simulink subsystem "Final_Project_PreRemoveOutputAdapter_20260527_143352"  (R2024a)
settings: Solver=VariableStepAuto  StartTime=0.0  StopTime=10.0  RelTol=1e-3
libraries: CarMaker4SL x42
settings Model: Creator=junho.lee  LastModifiedBy=hajin

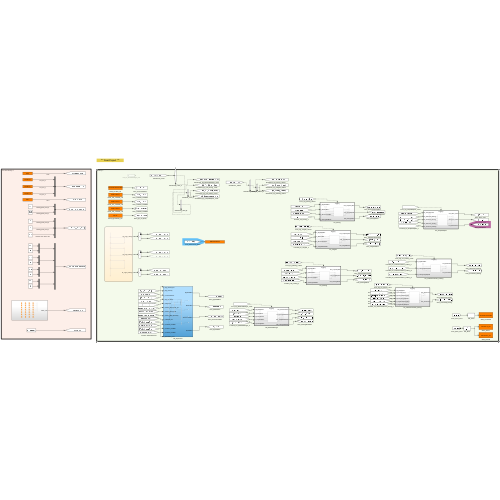
[thumbnail: Simulink's stored preview of the top-level diagram]
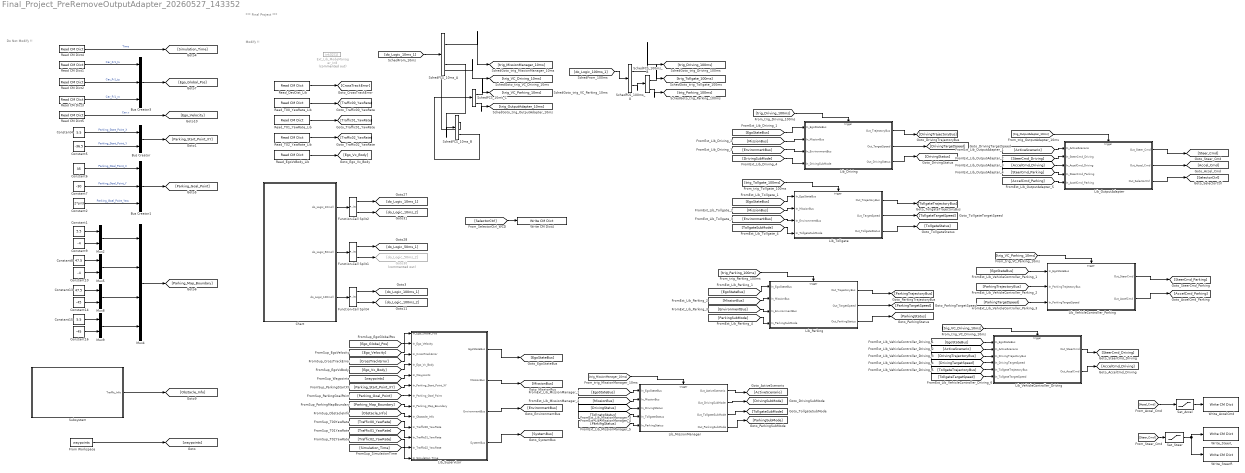
== system Final_Project_PreRemoveOutputAdapter_20260527_143352 ==
  note: Do Not Modify !!
  note: *** Final Project ***
  note: Modify !!
  Bus Creator : BusCreator  Inputs=2
  Bus Creator1 : BusCreator  Inputs=3
  Bus Creator3 : BusCreator  Inputs=3
  Chart : Stateflow chart  TreatAsAtomicUnit=on
  Constant1 : Constant  Value=5.5
  Constant10 : Constant  Value=-4
  Constant13 : Constant  Value=47.5
  Constant14 : Constant  Value=-45
  Constant15 : Constant  Value=5.5
  Constant16 : Constant  Value=-45
  Constant2 : Constant  Value=2*pi/3
  Constant4 : Constant  Value=5.5
  Constant5 : Constant  Value=-36.5
  Constant6 : Constant  Value=35
  Constant7 : Constant  Value=-30
  Constant8 : Constant  Value=47.5
  Constant9 : Constant  Value=-4
  Ext_Lib_ModeManager_In8 : Constant  Commented=on  Value=int32(1)  OutDataTypeStr=int32
  From Workspace : FromWorkspace  VariableName=waypoints
  Function-Call Split1 : FunctionCallSplit  IconShape=distinctive  NumOutputPorts=2  OutputPortLayout=default
  Function-Call Split2 : FunctionCallSplit  IconShape=distinctive  NumOutputPorts=2  OutputPortLayout=default
  Function-Call Split4 : FunctionCallSplit  IconShape=distinctive  NumOutputPorts=2  OutputPortLayout=default
  Goto30 : Goto  Commented=on  GotoTag=do_Logic_50ms_2
  Lib_Driving : Subsystem
  Lib_MissionManager : Subsystem
  Lib_OutputAdapter : Subsystem
  Lib_Parking : Subsystem
  Lib_Supervisor : Subsystem
  Lib_Tollgate : Subsystem
  Lib_VehicleController_Driving : Subsystem
  Lib_VehicleController_Parking : Subsystem
  Mux{2,5,8..9} (4 alike) : Mux  Inputs=2
  Mux4 : Mux
  Read CM Dict1 : CarMaker4SL/Read CM Dict  xname=Car.Fr1.tx  xsync=off  xstime=Inherited
  Read CM Dict2 : CarMaker4SL/Read CM Dict  xname=Car.Fr1.ty  xsync=off  xstime=Inherited
  Read CM Dict3 : CarMaker4SL/Read CM Dict  xname=Car.Fr1.rz  xsync=off  xstime=Inherited
  Read CM Dict4 : CarMaker4SL/Read CM Dict  xname=Time  xsync=off  xstime=Inherited
  Read CM Dict5 : CarMaker4SL/Read CM Dict  xname=Car.v  xsync=off  xstime=Inherited
  Read_DevDist_Lib : CarMaker4SL/Read CM Dict  xname=Car.Road.Path.DevDist  xsync=off  xstime=Inherited
  Read_EgoVxBody_Lib : CarMaker4SL/Read CM Dict  xname=Car.vx  xsync=off  xstime=Inherited
  Read_T00_YawRate_Lib : CarMaker4SL/Read CM Dict  xname=Traffic.T00.rzv  xsync=off  xstime=Inherited
  Read_T01_YawRate_Lib : CarMaker4SL/Read CM Dict  xname=Traffic.T01.rzv  xsync=off  xstime=Inherited
  Read_T02_YawRate_Lib : CarMaker4SL/Read CM Dict  xname=Traffic.T02.rzv  xsync=off  xstime=Inherited
  Sat_Accel : Saturate  UpperLimit=3.0  LowerLimit=-5.0
  Sat_Steer : Saturate  UpperLimit=pi/6  LowerLimit=-pi/6
  SchedFCS_100ms_A : FunctionCallSplit  NumOutputPorts=2
  SchedFCS_100ms_B : FunctionCallSplit  NumOutputPorts=2
  SchedFCS_10ms_A : FunctionCallSplit  NumOutputPorts=2
  SchedFCS_10ms_B : FunctionCallSplit  NumOutputPorts=2
  SchedFCS_10ms_C : FunctionCallSplit  NumOutputPorts=2
  Subsystem : Subsystem
  Write CM Dict4 : CarMaker4SL/Write CM Dict  xname=DM.SelectorCtrl  xsync=off
  Write_AccelCmd : CarMaker4SL/Write CM Dict  xname=AccelCtrl.DesiredAx  xsync=off
  Write_SteerL : CarMaker4SL/Write CM Dict  xname=Car.CFL.rz_ext  xsync=off
  Write_SteerR : CarMaker4SL/Write CM Dict  xname=Car.CFR.rz_ext  xsync=off
  wires:
  Constant13/1 -> Mux8/1
  Subsystem/1(Traffic_Info) -> [Obstacle_Info]
  Read CM Dict1/1 -> Bus Creator3/1  "Car_Fr1_tx"
  Read CM Dict3/1 -> Bus Creator3/3  "Car_Fr1_rz"
  Constant4/1 -> Bus Creator/1  "Parking_Start_Point_X"
  Chart/2(do_Logic_50ms()) -> Function-Call Split1/1
  Function-Call Split2/1 -> [do_Logic_10ms_1]
  Function-Call Split1/2 -> Goto30/1
  Read CM Dict4/1 -> [Simulation_Time]  "Time"
  Constant9/1 -> Mux2/2
  Bus Creator1/1 -> [Parking_Goal_Point]
  Mux8/1 -> Mux4/3
  Constant6/1 -> Bus Creator1/1  "Parking_Goal_Point_X"
  Constant1/1 -> Mux2/1
  Constant16/1 -> Mux9/2
  Read CM Dict2/1 -> Bus Creator3/2  "Car_Fr1_ty"
  Function-Call Split1/1 -> [do_Logic_50ms_1]
  Constant5/1 -> Bus Creator/2  "Parking_Start_Point_Y"
  Chart/1(do_Logic_10ms()) -> Function-Call Split2/1
  Constant7/1 -> Bus Creator1/2  "Parking_Goal_Point_Y"
  Read CM Dict5/1 -> [Ego_Velocity]  "Car.v"
  Constant15/1 -> Mux9/1
  Constant10/1 -> Mux5/2
  Bus Creator3/1 -> [Ego_Global_Pos]
  Constant14/1 -> Mux8/2
  Function-Call Split2/2 -> [do_Logic_10ms_2]
  Bus Creator/1 -> [Parking_Start_Point_XY]
  Mux9/1 -> Mux4/4
  Mux2/1 -> Mux4/1
  Mux4/1 -> [Parking_Map_Boundary]
  Constant8/1 -> Mux5/1
  Constant2/1 -> Bus Creator1/3  "Parking_Goal_Point_Yaw"
  Mux5/1 -> Mux4/2
  Chart/3(do_Logic_100ms()) -> Function-Call Split4/1
  Function-Call Split4/1 -> [do_Logic_100ms_1]
  Function-Call Split4/2 -> [do_Logic_100ms_2]
  From Workspace/1 -> [waypoints]
  [Accel_Cmd] -> Sat_Accel/1
  Sat_Accel/1 -> Write_AccelCmd/1
  [Steer_Cmd] -> Sat_Steer/1
  Sat_Steer/1 -> Write_SteerR/1, Write_SteerL/1
  Read_DevDist_Lib/1 -> [CrossTrackError]
  Read_T00_YawRate_Lib/1 -> [Traffic00_YawRate]
  Read_T01_YawRate_Lib/1 -> [Traffic01_YawRate]
  Read_T02_YawRate_Lib/1 -> [Traffic02_YawRate]
  Read_EgoVxBody_Lib/1 -> [Ego_Vx_Body]
  [Ego_Global_Pos] -> Lib_Supervisor/1(In_Ego_Global_Pos)
  [Ego_Velocity] -> Lib_Supervisor/2(In_Ego_Velocity)
  [CrossTrackError] -> Lib_Supervisor/3(In_CrossTrackError)
  [Ego_Vx_Body] -> Lib_Supervisor/4(In_Ego_Vx_Body)
  [waypoints] -> Lib_Supervisor/5(In_Waypoints)
  [Parking_Start_Point_XY] -> Lib_Supervisor/6(In_Parking_Start_Point_XY)
  [Parking_Goal_Point] -> Lib_Supervisor/7(In_Parking_Goal_Point)
  [Parking_Map_Boundary] -> Lib_Supervisor/8(In_Parking_Map_Boundary)
  [Obstacle_Info] -> Lib_Supervisor/9(In_Obstacle_Info)
  [Traffic00_YawRate] -> Lib_Supervisor/10(In_Traffic00_YawRate)
  [Traffic01_YawRate] -> Lib_Supervisor/11(In_Traffic01_YawRate)
  [Traffic02_YawRate] -> Lib_Supervisor/12(In_Traffic02_YawRate)
  [Simulation_Time] -> Lib_Supervisor/13(In_Simulation_Time)
  Lib_Supervisor/1(EgoStateBus) -> [EgoStateBus]
  Lib_Supervisor/2(MissionBus) -> [MissionBus]
  Lib_Supervisor/3(EnvironmentBus) -> [EnvironmentBus]
  Lib_Supervisor/4(SystemBus) -> [SystemBus]
  Lib_MissionManager/1(Out_ActiveScenario) -> [ActiveScenario]
  Lib_MissionManager/2(Out_DrivingSubMode) -> [DrivingSubMode]
  Lib_MissionManager/3(Out_TollgateSubMode) -> [TollgateSubMode]
  Lib_MissionManager/4(Out_ParkingSubMode) -> [ParkingSubMode]
  Lib_Driving/1(Out_TrajectoryBus) -> [DrivingTrajectoryBus]
  Lib_Driving/2(Out_TargetSpeed) -> [DrivingTargetSpeed]
  Lib_Driving/3(Out_DrivingStatus) -> [DrivingStatus]
  Lib_Tollgate/1(Out_TrajectoryBus) -> [TollgateTrajectoryBus]
  Lib_Tollgate/2(Out_TargetSpeed) -> [TollgateTargetSpeed]
  Lib_Tollgate/3(Out_TollgateStatus) -> [TollgateStatus]
  Lib_Parking/1(Out_TrajectoryBus) -> [ParkingTrajectoryBus]
  Lib_Parking/2(Out_TargetSpeed) -> [ParkingTargetSpeed]
  Lib_Parking/3(Out_ParkingStatus) -> [ParkingStatus]
  Lib_VehicleController_Driving/1(Out_SteerCmd) -> [SteerCmd_Driving]
  Lib_VehicleController_Driving/2(Out_AccelCmd) -> [AccelCmd_Driving]
  Lib_VehicleController_Parking/1(Out_SteerCmd) -> [SteerCmd_Parking]
  Lib_VehicleController_Parking/2(Out_AccelCmd) -> [AccelCmd_Parking]
  Lib_OutputAdapter/1(Out_Steer_Cmd) -> [Steer_Cmd]
  Lib_OutputAdapter/2(Out_Accel_Cmd) -> [Accel_Cmd]
  Lib_OutputAdapter/3(Out_SelectorCtrl) -> [SelectorCtrl]
  [EgoStateBus] -> Lib_MissionManager/1(In_EgoStateBus)
  [MissionBus] -> Lib_MissionManager/2(In_MissionBus)
  [DrivingStatus] -> Lib_MissionManager/3(In_DrivingStatus)
  [TollgateStatus] -> Lib_MissionManager/4(In_TollgateStatus)
  [ParkingStatus] -> Lib_MissionManager/5(In_ParkingStatus)
  [EgoStateBus] -> Lib_Driving/1(In_EgoStateBus)
  [MissionBus] -> Lib_Driving/2(In_MissionBus)
  [EnvironmentBus] -> Lib_Driving/3(In_EnvironmentBus)
  [DrivingSubMode] -> Lib_Driving/4(In_DrivingSubMode)
  [EgoStateBus] -> Lib_Tollgate/1(In_EgoStateBus)
  [MissionBus] -> Lib_Tollgate/2(In_MissionBus)
  [EnvironmentBus] -> Lib_Tollgate/3(In_EnvironmentBus)
  [TollgateSubMode] -> Lib_Tollgate/4(In_TollgateSubMode)
  [EgoStateBus] -> Lib_Parking/1(In_EgoStateBus)
  [MissionBus] -> Lib_Parking/2(In_MissionBus)
  [EnvironmentBus] -> Lib_Parking/3(In_EnvironmentBus)
  [ParkingSubMode] -> Lib_Parking/4(In_ParkingSubMode)
  [EgoStateBus] -> Lib_VehicleController_Driving/1(In_EgoStateBus)
  [ActiveScenario] -> Lib_VehicleController_Driving/2(In_ActiveScenario)
  [DrivingTrajectoryBus] -> Lib_VehicleController_Driving/3(In_DrivingTrajectoryBus)
  [DrivingTargetSpeed] -> Lib_VehicleController_Driving/4(In_DrivingTargetSpeed)
  [TollgateTrajectoryBus] -> Lib_VehicleController_Driving/5(In_TollgateTrajectoryBus)
  [TollgateTargetSpeed] -> Lib_VehicleController_Driving/6(In_TollgateTargetSpeed)
  [EgoStateBus] -> Lib_VehicleController_Parking/1(In_EgoStateBus)
  [ParkingTrajectoryBus] -> Lib_VehicleController_Parking/2(In_ParkingTrajectoryBus)
  [ParkingTargetSpeed] -> Lib_VehicleController_Parking/3(In_ParkingTargetSpeed)
  [ActiveScenario] -> Lib_OutputAdapter/1(In_ActiveScenario)
  [SteerCmd_Driving] -> Lib_OutputAdapter/2(In_SteerCmd_Driving)
  [AccelCmd_Driving] -> Lib_OutputAdapter/3(In_AccelCmd_Driving)
  [SteerCmd_Parking] -> Lib_OutputAdapter/4(In_SteerCmd_Parking)
  [AccelCmd_Parking] -> Lib_OutputAdapter/5(In_AccelCmd_Parking)
  [do_Logic_10ms_1] -> SchedFCS_10ms_A/1
  SchedFCS_10ms_A/1 -> [trig_MissionManager_10ms]
  SchedFCS_10ms_A/2 -> SchedFCS_10ms_B/1
  SchedFCS_10ms_B/1 -> [trig_VC_Driving_10ms]
  SchedFCS_10ms_B/2 -> SchedFCS_10ms_C/1
  SchedFCS_10ms_C/1 -> [trig_VC_Parking_10ms]
  SchedFCS_10ms_C/2 -> [trig_OutputAdapter_10ms]
  [do_Logic_100ms_1] -> SchedFCS_100ms_A/1
  SchedFCS_100ms_A/1 -> [trig_Driving_100ms]
  SchedFCS_100ms_A/2 -> SchedFCS_100ms_B/1
  SchedFCS_100ms_B/1 -> [trig_Tollgate_100ms]
  SchedFCS_100ms_B/2 -> [trig_Parking_100ms]
  [trig_MissionManager_10ms] -> Lib_MissionManager/Trigger
  [trig_VC_Driving_10ms] -> Lib_VehicleController_Driving/Trigger
  [trig_VC_Parking_10ms] -> Lib_VehicleController_Parking/Trigger
  [trig_OutputAdapter_10ms] -> Lib_OutputAdapter/Trigger
  [trig_Driving_100ms] -> Lib_Driving/Trigger
  [trig_Tollgate_100ms] -> Lib_Tollgate/Trigger
  [trig_Parking_100ms] -> Lib_Parking/Trigger
  [SelectorCtrl] -> Write CM Dict4/1

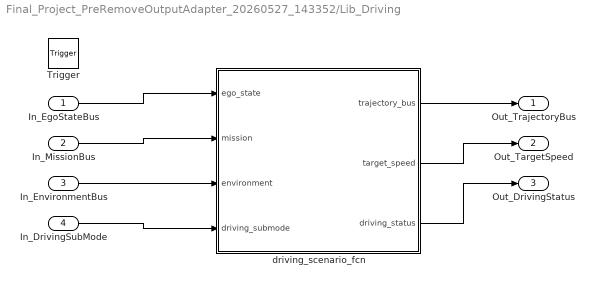
== system Final_Project_PreRemoveOutputAdapter_20260527_143352/Lib_Driving ==
  In_EgoStateBus : Inport
  In_MissionBus : Inport  Port=2
  In_EnvironmentBus : Inport  Port=3
  In_DrivingSubMode : Inport  Port=4
  Trigger : TriggerPort  TriggerType=function-call  VariantControl=(inherit)
  driving_scenario_fcn : MATLAB Function  TreatAsAtomicUnit=on
  Out_TrajectoryBus : Outport
  Out_TargetSpeed : Outport  Port=2
  Out_DrivingStatus : Outport  Port=3
  wires:
  In_EgoStateBus/1 -> driving_scenario_fcn/1(ego_state)
  In_MissionBus/1 -> driving_scenario_fcn/2(mission)
  In_EnvironmentBus/1 -> driving_scenario_fcn/3(environment)
  In_DrivingSubMode/1 -> driving_scenario_fcn/4(driving_submode)
  driving_scenario_fcn/1(trajectory_bus) -> Out_TrajectoryBus/1
  driving_scenario_fcn/2(target_speed) -> Out_TargetSpeed/1
  driving_scenario_fcn/3(driving_status) -> Out_DrivingStatus/1

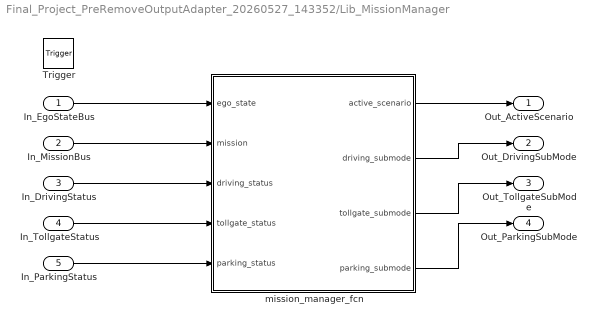
== system Final_Project_PreRemoveOutputAdapter_20260527_143352/Lib_MissionManager ==
  In_EgoStateBus : Inport
  In_MissionBus : Inport  Port=2
  In_DrivingStatus : Inport  Port=3
  In_TollgateStatus : Inport  Port=4
  In_ParkingStatus : Inport  Port=5
  Trigger : TriggerPort  TriggerType=function-call  VariantControl=(inherit)
  mission_manager_fcn : MATLAB Function  TreatAsAtomicUnit=on
  Out_ActiveScenario : Outport
  Out_DrivingSubMode : Outport  Port=2
  Out_TollgateSubMode : Outport  Port=3
  Out_ParkingSubMode : Outport  Port=4
  wires:
  In_EgoStateBus/1 -> mission_manager_fcn/1(ego_state)
  In_MissionBus/1 -> mission_manager_fcn/2(mission)
  In_DrivingStatus/1 -> mission_manager_fcn/3(driving_status)
  In_TollgateStatus/1 -> mission_manager_fcn/4(tollgate_status)
  In_ParkingStatus/1 -> mission_manager_fcn/5(parking_status)
  mission_manager_fcn/1(active_scenario) -> Out_ActiveScenario/1
  mission_manager_fcn/2(driving_submode) -> Out_DrivingSubMode/1
  mission_manager_fcn/3(tollgate_submode) -> Out_TollgateSubMode/1
  mission_manager_fcn/4(parking_submode) -> Out_ParkingSubMode/1

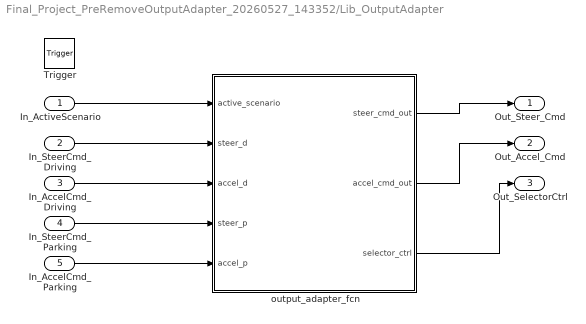
== system Final_Project_PreRemoveOutputAdapter_20260527_143352/Lib_OutputAdapter ==
  In_ActiveScenario : Inport
  In_SteerCmd_Driving : Inport  Port=2
  In_AccelCmd_Driving : Inport  Port=3
  In_SteerCmd_Parking : Inport  Port=4
  In_AccelCmd_Parking : Inport  Port=5
  Trigger : TriggerPort  TriggerType=function-call  VariantControl=(inherit)
  output_adapter_fcn : MATLAB Function  TreatAsAtomicUnit=on
  Out_Steer_Cmd : Outport
  Out_Accel_Cmd : Outport  Port=2
  Out_SelectorCtrl : Outport  Port=3
  wires:
  In_ActiveScenario/1 -> output_adapter_fcn/1(active_scenario)
  In_SteerCmd_Driving/1 -> output_adapter_fcn/2(steer_d)
  In_AccelCmd_Driving/1 -> output_adapter_fcn/3(accel_d)
  In_SteerCmd_Parking/1 -> output_adapter_fcn/4(steer_p)
  In_AccelCmd_Parking/1 -> output_adapter_fcn/5(accel_p)
  output_adapter_fcn/1(steer_cmd_out) -> Out_Steer_Cmd/1
  output_adapter_fcn/2(accel_cmd_out) -> Out_Accel_Cmd/1
  output_adapter_fcn/3(selector_ctrl) -> Out_SelectorCtrl/1

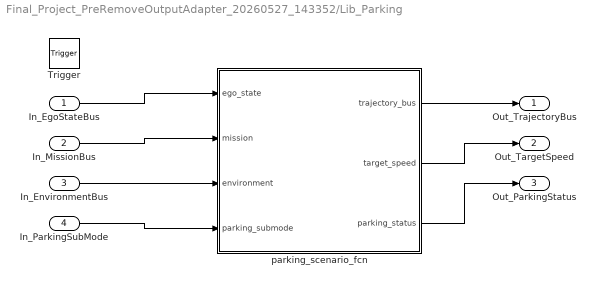
== system Final_Project_PreRemoveOutputAdapter_20260527_143352/Lib_Parking ==
  In_EgoStateBus : Inport
  In_MissionBus : Inport  Port=2
  In_EnvironmentBus : Inport  Port=3
  In_ParkingSubMode : Inport  Port=4
  Trigger : TriggerPort  TriggerType=function-call  VariantControl=(inherit)
  parking_scenario_fcn : MATLAB Function  TreatAsAtomicUnit=on
  Out_TrajectoryBus : Outport
  Out_TargetSpeed : Outport  Port=2
  Out_ParkingStatus : Outport  Port=3
  wires:
  In_EgoStateBus/1 -> parking_scenario_fcn/1(ego_state)
  In_MissionBus/1 -> parking_scenario_fcn/2(mission)
  In_EnvironmentBus/1 -> parking_scenario_fcn/3(environment)
  In_ParkingSubMode/1 -> parking_scenario_fcn/4(parking_submode)
  parking_scenario_fcn/1(trajectory_bus) -> Out_TrajectoryBus/1
  parking_scenario_fcn/2(target_speed) -> Out_TargetSpeed/1
  parking_scenario_fcn/3(parking_status) -> Out_ParkingStatus/1

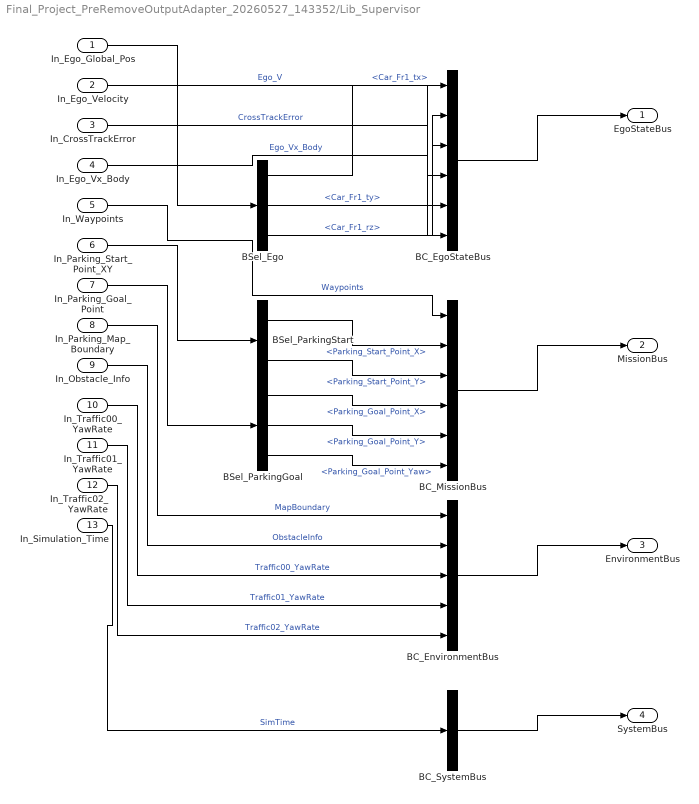
== system Final_Project_PreRemoveOutputAdapter_20260527_143352/Lib_Supervisor ==
  In_Ego_Global_Pos : Inport
  In_Ego_Velocity : Inport  Port=2
  In_CrossTrackError : Inport  Port=3
  In_Ego_Vx_Body : Inport  Port=4
  In_Waypoints : Inport  Port=5
  In_Parking_Start_Point_XY : Inport  Port=6
  In_Parking_Goal_Point : Inport  Port=7
  In_Parking_Map_Boundary : Inport  Port=8
  In_Obstacle_Info : Inport  Port=9
  In_Traffic00_YawRate : Inport  Port=10
  In_Traffic01_YawRate : Inport  Port=11
  In_Traffic02_YawRate : Inport  Port=12
  In_Simulation_Time : Inport  Port=13
  BC_EgoStateBus : BusCreator  Inputs=6
  BC_EnvironmentBus : BusCreator  Inputs=5
  BC_MissionBus : BusCreator  Inputs=6
  BC_SystemBus : BusCreator  Inputs=1
  BSel_Ego : BusSelector  OutputSignals=Car_Fr1_tx,Car_Fr1_ty,Car_Fr1_rz
  BSel_ParkingGoal : BusSelector  OutputSignals=Parking_Goal_Point_X,Parking_Goal_Point_Y,Parking_Goal_Point_Yaw
  BSel_ParkingStart : BusSelector  OutputSignals=Parking_Start_Point_X,Parking_Start_Point_Y
  EgoStateBus : Outport
  MissionBus : Outport  Port=2
  EnvironmentBus : Outport  Port=3
  SystemBus : Outport  Port=4
  wires:
  In_Ego_Global_Pos/1 -> BSel_Ego/1
  In_Parking_Start_Point_XY/1 -> BSel_ParkingStart/1
  In_Parking_Goal_Point/1 -> BSel_ParkingGoal/1
  BSel_Ego/1 -> BC_EgoStateBus/1  "<Car_Fr1_tx>"
  BSel_Ego/2 -> BC_EgoStateBus/2  "<Car_Fr1_ty>"
  BSel_Ego/3 -> BC_EgoStateBus/3  "<Car_Fr1_rz>"
  In_Ego_Velocity/1 -> BC_EgoStateBus/4  "Ego_V"
  In_CrossTrackError/1 -> BC_EgoStateBus/5  "CrossTrackError"
  In_Ego_Vx_Body/1 -> BC_EgoStateBus/6  "Ego_Vx_Body"
  In_Waypoints/1 -> BC_MissionBus/1  "Waypoints"
  BSel_ParkingStart/1 -> BC_MissionBus/2  "<Parking_Start_Point_X>"
  BSel_ParkingStart/2 -> BC_MissionBus/3  "<Parking_Start_Point_Y>"
  BSel_ParkingGoal/1 -> BC_MissionBus/4  "<Parking_Goal_Point_X>"
  BSel_ParkingGoal/2 -> BC_MissionBus/5  "<Parking_Goal_Point_Y>"
  BSel_ParkingGoal/3 -> BC_MissionBus/6  "<Parking_Goal_Point_Yaw>"
  In_Parking_Map_Boundary/1 -> BC_EnvironmentBus/1  "MapBoundary"
  In_Obstacle_Info/1 -> BC_EnvironmentBus/2  "ObstacleInfo"
  In_Traffic00_YawRate/1 -> BC_EnvironmentBus/3  "Traffic00_YawRate"
  In_Traffic01_YawRate/1 -> BC_EnvironmentBus/4  "Traffic01_YawRate"
  In_Traffic02_YawRate/1 -> BC_EnvironmentBus/5  "Traffic02_YawRate"
  In_Simulation_Time/1 -> BC_SystemBus/1  "SimTime"
  BC_EgoStateBus/1 -> EgoStateBus/1
  BC_MissionBus/1 -> MissionBus/1
  BC_EnvironmentBus/1 -> EnvironmentBus/1
  BC_SystemBus/1 -> SystemBus/1

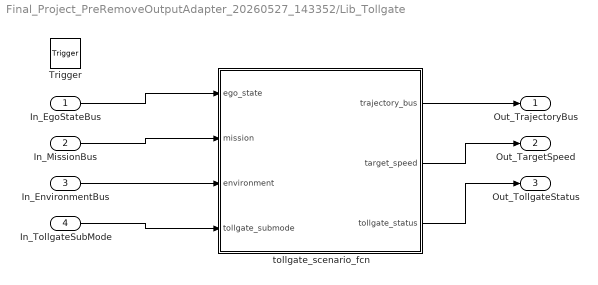
== system Final_Project_PreRemoveOutputAdapter_20260527_143352/Lib_Tollgate ==
  In_EgoStateBus : Inport
  In_MissionBus : Inport  Port=2
  In_EnvironmentBus : Inport  Port=3
  In_TollgateSubMode : Inport  Port=4
  Trigger : TriggerPort  TriggerType=function-call  VariantControl=(inherit)
  tollgate_scenario_fcn : MATLAB Function  TreatAsAtomicUnit=on
  Out_TrajectoryBus : Outport
  Out_TargetSpeed : Outport  Port=2
  Out_TollgateStatus : Outport  Port=3
  wires:
  In_EgoStateBus/1 -> tollgate_scenario_fcn/1(ego_state)
  In_MissionBus/1 -> tollgate_scenario_fcn/2(mission)
  In_EnvironmentBus/1 -> tollgate_scenario_fcn/3(environment)
  In_TollgateSubMode/1 -> tollgate_scenario_fcn/4(tollgate_submode)
  tollgate_scenario_fcn/1(trajectory_bus) -> Out_TrajectoryBus/1
  tollgate_scenario_fcn/2(target_speed) -> Out_TargetSpeed/1
  tollgate_scenario_fcn/3(tollgate_status) -> Out_TollgateStatus/1

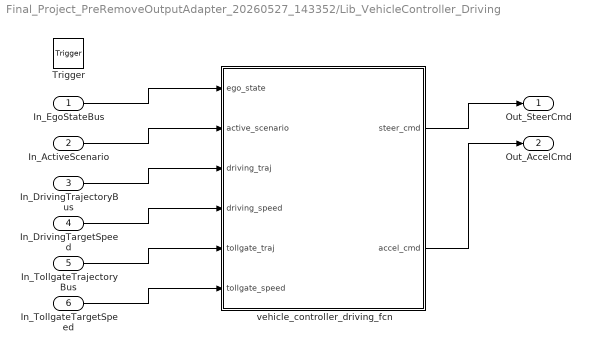
== system Final_Project_PreRemoveOutputAdapter_20260527_143352/Lib_VehicleController_Driving ==
  In_EgoStateBus : Inport
  In_ActiveScenario : Inport  Port=2
  In_DrivingTrajectoryBus : Inport  Port=3
  In_DrivingTargetSpeed : Inport  Port=4
  In_TollgateTrajectoryBus : Inport  Port=5
  In_TollgateTargetSpeed : Inport  Port=6
  Trigger : TriggerPort  TriggerType=function-call  VariantControl=(inherit)
  vehicle_controller_driving_fcn : MATLAB Function  TreatAsAtomicUnit=on
  Out_SteerCmd : Outport
  Out_AccelCmd : Outport  Port=2
  wires:
  In_EgoStateBus/1 -> vehicle_controller_driving_fcn/1(ego_state)
  In_ActiveScenario/1 -> vehicle_controller_driving_fcn/2(active_scenario)
  In_DrivingTrajectoryBus/1 -> vehicle_controller_driving_fcn/3(driving_traj)
  In_DrivingTargetSpeed/1 -> vehicle_controller_driving_fcn/4(driving_speed)
  In_TollgateTrajectoryBus/1 -> vehicle_controller_driving_fcn/5(tollgate_traj)
  In_TollgateTargetSpeed/1 -> vehicle_controller_driving_fcn/6(tollgate_speed)
  vehicle_controller_driving_fcn/1(steer_cmd) -> Out_SteerCmd/1
  vehicle_controller_driving_fcn/2(accel_cmd) -> Out_AccelCmd/1

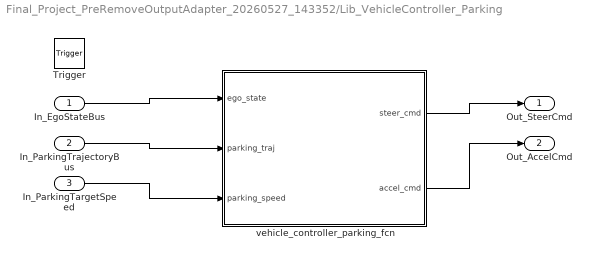
== system Final_Project_PreRemoveOutputAdapter_20260527_143352/Lib_VehicleController_Parking ==
  In_EgoStateBus : Inport
  In_ParkingTrajectoryBus : Inport  Port=2
  In_ParkingTargetSpeed : Inport  Port=3
  Trigger : TriggerPort  TriggerType=function-call  VariantControl=(inherit)
  vehicle_controller_parking_fcn : MATLAB Function  TreatAsAtomicUnit=on
  Out_SteerCmd : Outport
  Out_AccelCmd : Outport  Port=2
  wires:
  In_EgoStateBus/1 -> vehicle_controller_parking_fcn/1(ego_state)
  In_ParkingTrajectoryBus/1 -> vehicle_controller_parking_fcn/2(parking_traj)
  In_ParkingTargetSpeed/1 -> vehicle_controller_parking_fcn/3(parking_speed)
  vehicle_controller_parking_fcn/1(steer_cmd) -> Out_SteerCmd/1
  vehicle_controller_parking_fcn/2(accel_cmd) -> Out_AccelCmd/1

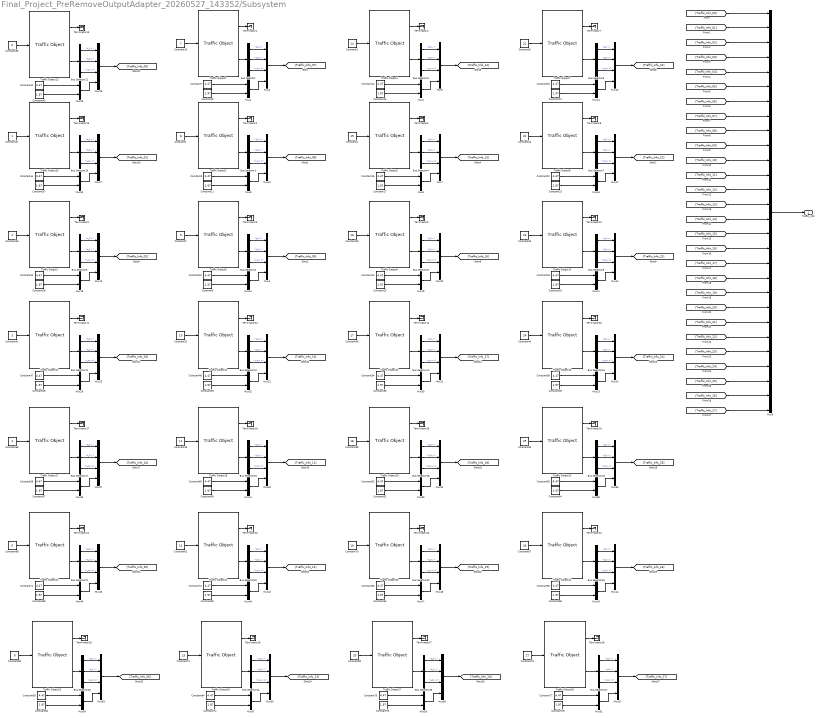
== system Final_Project_PreRemoveOutputAdapter_20260527_143352/Subsystem ==
  Bus Selector{,1..27} (28 alike) : BusSelector  OutputSignals=t_0 x,t_0 y,r_zyx z
  Constant1 : Constant  Value=8
  Constant10 : Constant  Value=7
  Constant{5,8,11,13,15,17,19,21,23,28,33,35,37,39,43,45,50,52,54,57,62,64,66,69,74,76,78,81} (28 alike) : Constant  Value=1.97
  Constant{7,9,12,14,16,18,20,22,30..31,34,38,42,44,47..48,51,53,59..60,63,65,71..72,75,77,83..84} (28 alike) : Constant  Value=4.47
  Constant2 : Constant  Value=9
  Constant24 : Constant  Value=22
  Constant25 : Constant  Value=23
  Constant26 : Constant  Value=2
  Constant27 : Constant
  Constant29 : Constant  Value=16
  Constant3 : Constant  Value=14
  Constant32 : Constant  Value=10
  Constant36 : Constant  Value=0
  Constant4 : Constant  Value=15
  Constant40 : Constant  Value=24
  Constant41 : Constant  Value=3
  Constant46 : Constant  Value=17
  Constant49 : Constant  Value=11
  Constant55 : Constant  Value=25
  Constant56 : Constant  Value=4
  Constant58 : Constant  Value=18
  Constant6 : Constant  Value=21
  Constant61 : Constant  Value=12
  Constant67 : Constant  Value=26
  Constant68 : Constant  Value=5
  Constant70 : Constant  Value=19
  Constant73 : Constant  Value=13
  Constant79 : Constant  Value=27
  Constant80 : Constant  Value=6
  Constant82 : Constant  Value=20
  Mux{1,4,6,8,11,14,16,18..19,21,23,26,28,30,32..33,35,38..39,41,43,46..47,49,51,54..55,57} (28 alike) : Mux  Inputs=2
  Mux{2..3,5,7,10,12..13,15,17,20,22,24..25,27,29,31,34,36..37,40,42,44..45,48,50,52..53,56} (28 alike) : Mux
  Mux9 : Mux  Inputs=28
  Terminator{1..28} (28 alike) : Terminator
  Traffic Object1 : CarMaker4SL/Traffic Object  xname=T07  ximode=Traffic Id  xstime=Inherited
      settings: SourceProductName=CarMaker4SL
  Traffic Object10 : CarMaker4SL/Traffic Object  xname=T23  ximode=Traffic Id  xstime=Inherited
      settings: SourceProductName=CarMaker4SL
  Traffic Object11 : CarMaker4SL/Traffic Object  xname=T03  ximode=Traffic Id  xstime=Inherited
      settings: SourceProductName=CarMaker4SL
  Traffic Object12 : CarMaker4SL/Traffic Object  xname=T10  ximode=Traffic Id  xstime=Inherited
      settings: SourceProductName=CarMaker4SL
  Traffic Object13 : CarMaker4SL/Traffic Object  xname=T00  ximode=Traffic Id  xstime=Inherited
      settings: SourceProductName=CarMaker4SL
  Traffic Object14 : CarMaker4SL/Traffic Object  xname=T17  ximode=Traffic Id  xstime=Inherited
      settings: SourceProductName=CarMaker4SL
  Traffic Object15 : CarMaker4SL/Traffic Object  xname=T01  ximode=Traffic Id  xstime=Inherited
      settings: SourceProductName=CarMaker4SL
  Traffic Object16 : CarMaker4SL/Traffic Object  xname=T24  ximode=Traffic Id  xstime=Inherited
      settings: SourceProductName=CarMaker4SL
  Traffic Object17 : CarMaker4SL/Traffic Object  xname=T04  ximode=Traffic Id  xstime=Inherited
      settings: SourceProductName=CarMaker4SL
  Traffic Object18 : CarMaker4SL/Traffic Object  xname=T11  ximode=Traffic Id  xstime=Inherited
      settings: SourceProductName=CarMaker4SL
  Traffic Object19 : CarMaker4SL/Traffic Object  xname=T18  ximode=Traffic Id  xstime=Inherited
      settings: SourceProductName=CarMaker4SL
  Traffic Object2 : CarMaker4SL/Traffic Object  xname=T08  ximode=Traffic Id  xstime=Inherited
      settings: SourceProductName=CarMaker4SL
  Traffic Object20 : CarMaker4SL/Traffic Object  xname=T25  ximode=Traffic Id  xstime=Inherited
      settings: SourceProductName=CarMaker4SL
  Traffic Object21 : CarMaker4SL/Traffic Object  xname=T05  ximode=Traffic Id  xstime=Inherited
      settings: SourceProductName=CarMaker4SL
  Traffic Object22 : CarMaker4SL/Traffic Object  xname=T12  ximode=Traffic Id  xstime=Inherited
      settings: SourceProductName=CarMaker4SL
  Traffic Object23 : CarMaker4SL/Traffic Object  xname=T19  ximode=Traffic Id  xstime=Inherited
      settings: SourceProductName=CarMaker4SL
  Traffic Object24 : CarMaker4SL/Traffic Object  xname=T26  ximode=Traffic Id  xstime=Inherited
      settings: SourceProductName=CarMaker4SL
  Traffic Object25 : CarMaker4SL/Traffic Object  xname=T06  ximode=Traffic Id  xstime=Inherited
      settings: SourceProductName=CarMaker4SL
  Traffic Object26 : CarMaker4SL/Traffic Object  xname=T13  ximode=Traffic Id  xstime=Inherited
      settings: SourceProductName=CarMaker4SL
  Traffic Object27 : CarMaker4SL/Traffic Object  xname=T20  ximode=Traffic Id  xstime=Inherited
      settings: SourceProductName=CarMaker4SL
  Traffic Object28 : CarMaker4SL/Traffic Object  xname=T27  ximode=Traffic Id  xstime=Inherited
      settings: SourceProductName=CarMaker4SL
  Traffic Object3 : CarMaker4SL/Traffic Object  xname=T02  ximode=Traffic Id  xstime=Inherited
      settings: SourceProductName=CarMaker4SL
  Traffic Object4 : CarMaker4SL/Traffic Object  xname=T14  ximode=Traffic Id  xstime=Inherited
      settings: SourceProductName=CarMaker4SL
  Traffic Object5 : CarMaker4SL/Traffic Object  xname=T15  ximode=Traffic Id  xstime=Inherited
      settings: SourceProductName=CarMaker4SL
  Traffic Object6 : CarMaker4SL/Traffic Object  xname=T09  ximode=Traffic Id  xstime=Inherited
      settings: SourceProductName=CarMaker4SL
  Traffic Object7 : CarMaker4SL/Traffic Object  xname=T21  ximode=Traffic Id  xstime=Inherited
      settings: SourceProductName=CarMaker4SL
  Traffic Object8 : CarMaker4SL/Traffic Object  xname=T22  ximode=Traffic Id  xstime=Inherited
      settings: SourceProductName=CarMaker4SL
  Traffic Object9 : CarMaker4SL/Traffic Object  xname=T16  ximode=Traffic Id  xstime=Inherited
      settings: SourceProductName=CarMaker4SL
  Traffic_Info : Outport
  wires:
  [Traffic_Info_21] -> Mux9/22
  [Traffic_Info_27] -> Mux9/28
  [Traffic_Info_26] -> Mux9/27
  [Traffic_Info_22] -> Mux9/23
  [Traffic_Info_25] -> Mux9/26
  [Traffic_Info_24] -> Mux9/25
  [Traffic_Info_23] -> Mux9/24
  [Traffic_Info_14] -> Mux9/15
  [Traffic_Info_20] -> Mux9/21
  [Traffic_Info_19] -> Mux9/20
  [Traffic_Info_15] -> Mux9/16
  [Traffic_Info_18] -> Mux9/19
  [Traffic_Info_17] -> Mux9/18
  [Traffic_Info_16] -> Mux9/17
  [Traffic_Info_07] -> Mux9/8
  [Traffic_Info_13] -> Mux9/14
  [Traffic_Info_12] -> Mux9/13
  [Traffic_Info_08] -> Mux9/9
  [Traffic_Info_11] -> Mux9/12
  [Traffic_Info_10] -> Mux9/11
  [Traffic_Info_09] -> Mux9/10
  Constant84/1 -> Mux57/1
  Traffic Object27/2 -> Bus Selector26/1
  Constant83/1 -> Mux54/1
  Mux54/1 -> Mux53/4
  Bus Selector25/1 -> Mux53/1  "<t_0 x>"
  Bus Selector26/2 -> Mux56/2  "<t_0 y>"
  Mux56/1 -> [Traffic_Info_20]
  Constant73/1 -> Traffic Object26/1
  Bus Selector25/3 -> Mux53/3  "<r_zyx z>"
  Constant82/1 -> Traffic Object27/1
  Mux53/1 -> [Traffic_Info_06]
  Traffic Object28/1 -> Terminator28/1
  Traffic Object25/1 -> Terminator25/1
  Traffic Object25/2 -> Bus Selector25/1
  Constant81/1 -> Mux54/2
  Bus Selector24/3 -> Mux50/3  "<r_zyx z>"
  Traffic Object26/1 -> Terminator26/1
  Bus Selector24/1 -> Mux50/1  "<t_0 x>"
  Traffic Object27/1 -> Terminator27/1
  Traffic Object26/2 -> Bus Selector24/1
  Mux57/1 -> Mux50/4
  Bus Selector26/1 -> Mux56/1  "<t_0 x>"
  Constant76/1 -> Mux55/2
  Bus Selector24/2 -> Mux50/2  "<t_0 y>"
  Bus Selector27/2 -> Mux52/2  "<t_0 y>"
  Mux50/1 -> [Traffic_Info_13]
  Bus Selector25/2 -> Mux53/2  "<t_0 y>"
  Constant80/1 -> Traffic Object25/1
  Constant75/1 -> Mux55/1
  Bus Selector26/3 -> Mux56/3  "<r_zyx z>"
  Mux55/1 -> Mux56/4
  Constant74/1 -> Mux57/2
  Mux51/1 -> Mux52/4
  Bus Selector27/3 -> Mux52/3  "<r_zyx z>"
  Constant77/1 -> Mux51/1
  Traffic Object28/2 -> Bus Selector27/1
  Constant78/1 -> Mux51/2
  Bus Selector27/1 -> Mux52/1  "<t_0 x>"
  Mux52/1 -> [Traffic_Info_27]
  Constant79/1 -> Traffic Object28/1
  Constant72/1 -> Mux49/1
  Traffic Object23/2 -> Bus Selector22/1
  Constant71/1 -> Mux46/1
  Mux46/1 -> Mux45/4
  Bus Selector21/1 -> Mux45/1  "<t_0 x>"
  Bus Selector22/2 -> Mux48/2  "<t_0 y>"
  Mux48/1 -> [Traffic_Info_19]
  Constant61/1 -> Traffic Object22/1
  Bus Selector21/3 -> Mux45/3  "<r_zyx z>"
  Constant70/1 -> Traffic Object23/1
  Mux45/1 -> [Traffic_Info_05]
  Traffic Object24/1 -> Terminator24/1
  Traffic Object21/1 -> Terminator21/1
  Traffic Object21/2 -> Bus Selector21/1
  Constant69/1 -> Mux46/2
  Bus Selector20/3 -> Mux42/3  "<r_zyx z>"
  Traffic Object22/1 -> Terminator22/1
  Bus Selector20/1 -> Mux42/1  "<t_0 x>"
  Traffic Object23/1 -> Terminator23/1
  Traffic Object22/2 -> Bus Selector20/1
  Mux49/1 -> Mux42/4
  Bus Selector22/1 -> Mux48/1  "<t_0 x>"
  Constant64/1 -> Mux47/2
  Bus Selector20/2 -> Mux42/2  "<t_0 y>"
  Bus Selector23/2 -> Mux44/2  "<t_0 y>"
  Mux42/1 -> [Traffic_Info_12]
  Bus Selector21/2 -> Mux45/2  "<t_0 y>"
  Constant68/1 -> Traffic Object21/1
  Constant63/1 -> Mux47/1
  Bus Selector22/3 -> Mux48/3  "<r_zyx z>"
  Mux47/1 -> Mux48/4
  Constant62/1 -> Mux49/2
  Mux43/1 -> Mux44/4
  Bus Selector23/3 -> Mux44/3  "<r_zyx z>"
  Constant65/1 -> Mux43/1
  Traffic Object24/2 -> Bus Selector23/1
  Constant66/1 -> Mux43/2
  Bus Selector23/1 -> Mux44/1  "<t_0 x>"
  Mux44/1 -> [Traffic_Info_26]
  Constant67/1 -> Traffic Object24/1
  Constant60/1 -> Mux41/1
  Traffic Object19/2 -> Bus Selector18/1
  Constant59/1 -> Mux38/1
  Mux38/1 -> Mux37/4
  Bus Selector17/1 -> Mux37/1  "<t_0 x>"
  Bus Selector18/2 -> Mux40/2  "<t_0 y>"
  Mux40/1 -> [Traffic_Info_18]
  Constant49/1 -> Traffic Object18/1
  Bus Selector17/3 -> Mux37/3  "<r_zyx z>"
  Constant58/1 -> Traffic Object19/1
  Mux37/1 -> [Traffic_Info_04]
  Traffic Object20/1 -> Terminator20/1
  Traffic Object17/1 -> Terminator17/1
  Traffic Object17/2 -> Bus Selector17/1
  Constant57/1 -> Mux38/2
  Bus Selector16/3 -> Mux34/3  "<r_zyx z>"
  Traffic Object18/1 -> Terminator18/1
  Bus Selector16/1 -> Mux34/1  "<t_0 x>"
  Traffic Object19/1 -> Terminator19/1
  Traffic Object18/2 -> Bus Selector16/1
  Mux41/1 -> Mux34/4
  Bus Selector18/1 -> Mux40/1  "<t_0 x>"
  Constant52/1 -> Mux39/2
  Bus Selector16/2 -> Mux34/2  "<t_0 y>"
  Bus Selector19/2 -> Mux36/2  "<t_0 y>"
  Mux34/1 -> [Traffic_Info_11]
  Bus Selector17/2 -> Mux37/2  "<t_0 y>"
  Constant56/1 -> Traffic Object17/1
  Constant51/1 -> Mux39/1
  Bus Selector18/3 -> Mux40/3  "<r_zyx z>"
  Mux39/1 -> Mux40/4
  Constant50/1 -> Mux41/2
  Mux35/1 -> Mux36/4
  Bus Selector19/3 -> Mux36/3  "<r_zyx z>"
  Constant53/1 -> Mux35/1
  Traffic Object20/2 -> Bus Selector19/1
  Constant54/1 -> Mux35/2
  Bus Selector19/1 -> Mux36/1  "<t_0 x>"
  Mux36/1 -> [Traffic_Info_25]
  Constant55/1 -> Traffic Object20/1
  Constant48/1 -> Mux32/1
  Traffic Object14/2 -> Bus Selector14/1
  Constant47/1 -> Mux28/1
  Mux28/1 -> Mux25/4
  Bus Selector11/1 -> Mux25/1  "<t_0 x>"
  Bus Selector14/2 -> Mux31/2  "<t_0 y>"
  Mux31/1 -> [Traffic_Info_17]
  Constant32/1 -> Traffic Object12/1
  Bus Selector11/3 -> Mux25/3  "<r_zyx z>"
  Constant46/1 -> Traffic Object14/1
  Mux25/1 -> [Traffic_Info_03]
  Traffic Object16/1 -> Terminator16/1
  Traffic Object11/1 -> Terminator11/1
  Traffic Object11/2 -> Bus Selector11/1
  Constant45/1 -> Mux28/2
  Bus Selector10/3 -> Mux22/3  "<r_zyx z>"
  Traffic Object12/1 -> Terminator12/1
  Bus Selector10/1 -> Mux22/1  "<t_0 x>"
  Traffic Object14/1 -> Terminator14/1
  Traffic Object12/2 -> Bus Selector10/1
  Mux32/1 -> Mux22/4
  Bus Selector14/1 -> Mux31/1  "<t_0 x>"
  Constant35/1 -> Mux30/2
  Bus Selector10/2 -> Mux22/2  "<t_0 y>"
  Bus Selector15/2 -> Mux24/2  "<t_0 y>"
  Mux22/1 -> [Traffic_Info_10]
  Bus Selector11/2 -> Mux25/2  "<t_0 y>"
  Constant41/1 -> Traffic Object11/1
  Constant34/1 -> Mux30/1
  Bus Selector14/3 -> Mux31/3  "<r_zyx z>"
  Mux30/1 -> Mux31/4
  Constant33/1 -> Mux32/2
  Mux23/1 -> Mux24/4
  Bus Selector15/3 -> Mux24/3  "<r_zyx z>"
  Constant38/1 -> Mux23/1
  Traffic Object16/2 -> Bus Selector15/1
  Constant39/1 -> Mux23/2
  Bus Selector15/1 -> Mux24/1  "<t_0 x>"
  Mux24/1 -> [Traffic_Info_24]
  Constant40/1 -> Traffic Object16/1
  Constant31/1 -> Mux21/1
  Traffic Object9/2 -> Bus Selector8/1
  Constant30/1 -> Mux18/1
  Mux18/1 -> Mux13/4
  Bus Selector5/1 -> Mux13/1  "<t_0 x>"
  Bus Selector8/2 -> Mux20/2  "<t_0 y>"
  Mux20/1 -> [Traffic_Info_16]
  Constant2/1 -> Traffic Object6/1
  Bus Selector5/3 -> Mux13/3  "<r_zyx z>"
  Constant29/1 -> Traffic Object9/1
  Mux13/1 -> [Traffic_Info_02]
  Traffic Object10/1 -> Terminator10/1
  Traffic Object3/1 -> Terminator3/1
  Traffic Object3/2 -> Bus Selector5/1
  Constant28/1 -> Mux18/2
  Bus Selector2/3 -> Mux3/3  "<r_zyx z>"
  Traffic Object6/1 -> Terminator6/1
  Bus Selector2/1 -> Mux3/1  "<t_0 x>"
  Traffic Object9/1 -> Terminator9/1
  Traffic Object6/2 -> Bus Selector2/1
  Mux21/1 -> Mux3/4
  Bus Selector8/1 -> Mux20/1  "<t_0 x>"
  Constant13/1 -> Mux19/2
  Bus Selector2/2 -> Mux3/2  "<t_0 y>"
  Bus Selector9/2 -> Mux12/2  "<t_0 y>"
  Mux3/1 -> [Traffic_Info_09]
  Bus Selector5/2 -> Mux13/2  "<t_0 y>"
  Constant26/1 -> Traffic Object3/1
  Constant12/1 -> Mux19/1
  Bus Selector8/3 -> Mux20/3  "<r_zyx z>"
  Mux19/1 -> Mux20/4
  Constant5/1 -> Mux21/2
  Mux11/1 -> Mux12/4
  Bus Selector9/3 -> Mux12/3  "<r_zyx z>"
  Constant18/1 -> Mux11/1
  Traffic Object10/2 -> Bus Selector9/1
  Constant19/1 -> Mux11/2
  Bus Selector9/1 -> Mux12/1  "<t_0 x>"
  Mux12/1 -> [Traffic_Info_23]
  Constant25/1 -> Traffic Object10/1
  Constant27/1 -> Traffic Object15/1
  Bus Selector12/3 -> Mux29/3  "<r_zyx z>"
  Mux29/1 -> [Traffic_Info_00]
  Constant43/1 -> Mux26/2
  Bus Selector13/2 -> Mux27/2  "<t_0 y>"
  Bus Selector13/3 -> Mux27/3  "<r_zyx z>"
  Mux33/1 -> Mux27/4
  Bus Selector13/1 -> Mux27/1  "<t_0 x>"
  Constant44/1 -> Mux33/1
  Bus Selector12/2 -> Mux29/2  "<t_0 y>"
  Traffic Object15/1 -> Terminator15/1
  Traffic Object13/1 -> Terminator13/1
  Traffic Object15/2 -> Bus Selector13/1
  Mux27/1 -> [Traffic_Info_01]
  Constant42/1 -> Mux26/1
  Constant36/1 -> Traffic Object13/1
  Bus Selector12/1 -> Mux29/1  "<t_0 x>"
  Mux26/1 -> Mux29/4
  Traffic Object13/2 -> Bus Selector12/1
  Constant37/1 -> Mux33/2
  Constant24/1 -> Traffic Object8/1
  Traffic Object8/1 -> Terminator8/1
  Bus Selector7/2 -> Mux17/2  "<t_0 y>"
  Mux17/1 -> [Traffic_Info_22]
  Bus Selector7/1 -> Mux17/1  "<t_0 x>"
  Bus Selector7/3 -> Mux17/3  "<r_zyx z>"
  Traffic Object8/2 -> Bus Selector7/1
  Constant23/1 -> Mux16/2
  Constant22/1 -> Mux16/1
  Mux16/1 -> Mux17/4
  Mux14/1 -> Mux15/4
  Constant20/1 -> Mux14/1
  Constant21/1 -> Mux14/2
  Mux6/1 -> Mux7/4
  Constant16/1 -> Mux6/1
  Constant17/1 -> Mux6/2
  Mux4/1 -> Mux5/4
  Constant14/1 -> Mux4/1
  Constant15/1 -> Mux4/2
  Mux8/1 -> Mux10/4
  Constant9/1 -> Mux8/1
  Constant11/1 -> Mux8/2
  Constant7/1 -> Mux1/1
  Mux1/1 -> Mux2/4
  Constant8/1 -> Mux1/2
  [Traffic_Info_03] -> Mux9/4
  [Traffic_Info_04] -> Mux9/5
  [Traffic_Info_05] -> Mux9/6
  [Traffic_Info_06] -> Mux9/7
  [Traffic_Info_02] -> Mux9/3
  Mux9/1 -> Traffic_Info/1
  [Traffic_Info_01] -> Mux9/2
  [Traffic_Info_00] -> Mux9/1
  Mux2/1 -> [Traffic_Info_07]
  Traffic Object7/2 -> Bus Selector6/1
  Bus Selector6/3 -> Mux15/3  "<r_zyx z>"
  Bus Selector6/1 -> Mux15/1  "<t_0 x>"
  Mux15/1 -> [Traffic_Info_21]
  Bus Selector6/2 -> Mux15/2  "<t_0 y>"
  Traffic Object5/2 -> Bus Selector4/1
  Bus Selector4/3 -> Mux7/3  "<r_zyx z>"
  Bus Selector4/1 -> Mux7/1  "<t_0 x>"
  Mux7/1 -> [Traffic_Info_15]
  Bus Selector4/2 -> Mux7/2  "<t_0 y>"
  Traffic Object4/2 -> Bus Selector3/1
  Bus Selector3/3 -> Mux5/3  "<r_zyx z>"
  Bus Selector3/1 -> Mux5/1  "<t_0 x>"
  Mux5/1 -> [Traffic_Info_14]
  Bus Selector3/2 -> Mux5/2  "<t_0 y>"
  Traffic Object2/2 -> Bus Selector1/1
  Bus Selector1/3 -> Mux10/3  "<r_zyx z>"
  Bus Selector1/1 -> Mux10/1  "<t_0 x>"
  Mux10/1 -> [Traffic_Info_08]
  Bus Selector1/2 -> Mux10/2  "<t_0 y>"
  Bus Selector/3 -> Mux2/3  "<r_zyx z>"
  Bus Selector/2 -> Mux2/2  "<t_0 y>"
  Bus Selector/1 -> Mux2/1  "<t_0 x>"
  Traffic Object1/2 -> Bus Selector/1
  Traffic Object7/1 -> Terminator7/1
  Constant6/1 -> Traffic Object7/1
  Traffic Object5/1 -> Terminator5/1
  Constant4/1 -> Traffic Object5/1
  Constant3/1 -> Traffic Object4/1
  Traffic Object4/1 -> Terminator4/1
  Constant1/1 -> Traffic Object2/1
  Traffic Object2/1 -> Terminator2/1
  Traffic Object1/1 -> Terminator1/1
  Constant10/1 -> Traffic Object1/1

== matlab function Final_Project_PreRemoveOutputAdapter_20260527_143352/Lib_VehicleController_Parking/vehicle_controller_parking_fcn ==
  data: ego_state input; steer_cmd output; parking_traj input; parking_speed input; accel_cmd output
function [steer_cmd, accel_cmd] = wrapper(ego_state, parking_traj, parking_speed)
%#codegen
% Wrapper: edit functions/vehicle_controller_parking_fcn.m, NOT this block
[steer_cmd, accel_cmd] = vehicle_controller_parking_fcn(ego_state, parking_traj, parking_speed);
end

== matlab function Final_Project_PreRemoveOutputAdapter_20260527_143352/Lib_OutputAdapter/output_adapter_fcn ==
  data: active_scenario input; steer_cmd_out output; steer_d input; accel_d input; steer_p input; accel_p input; accel_cmd_out output; selector_ctrl output
function [steer_cmd_out, accel_cmd_out, selector_ctrl] = wrapper(active_scenario, steer_d, accel_d, steer_p, accel_p)
%#codegen
% Wrapper: edit functions/output_adapter_fcn.m, NOT this block
[steer_cmd_out, accel_cmd_out, selector_ctrl] = output_adapter_fcn(active_scenario, steer_d, accel_d, steer_p, accel_p);
end

== stateflow chart Final_Project_PreRemoveOutputAdapter_20260527_143352/Chart ==
  (default) -> (junction 1)
  (junction 1) -> (junction 3) [order 1] : [mod(i,10) == 0]
      | {do_Logic_10ms;}
  (junction 1) -> (junction 7) [order 2]
  (junction 3) -> (junction 5)
  (junction 5) -> (junction 7)
  (junction 7) -> (junction 10)
  (junction 10) -> (junction 12) [order 1] : [mod(i, 50) == 0]
      | {do_Logic_50ms;}
  (junction 10) -> (junction 18) [order 2]
  (junction 12) -> (junction 16)
  (junction 16) -> (junction 18)
  (junction 18) -> (junction 25)
  (junction 25) -> (junction 27) [order 1] : [mod(i,100) == 0]
      | {do_Logic_100ms;}
  (junction 25) -> (junction 21) [order 2]
  (junction 27) -> (junction 29) : {i = 0;}
  (junction 29) -> (junction 21)
  (junction 21) -> (junction 32) : {i = i +1;}
  data: i local =0
  events: do_Logic_10ms output FUNCTION_CALL_EVENT; do_Logic_50ms output FUNCTION_CALL_EVENT; do_Logic_100ms output FUNCTION_CALL_EVENT

== matlab function Final_Project_PreRemoveOutputAdapter_20260527_143352/Lib_Driving/driving_scenario_fcn ==
  data: ego_state input; trajectory_bus output; mission input; environment input; driving_submode input; target_speed output; driving_status output
function [trajectory_bus, target_speed, driving_status] = wrapper(ego_state, mission, environment, driving_submode)
%#codegen
% Wrapper: edit functions/driving_scenario_fcn.m, NOT this block
[trajectory_bus, target_speed, driving_status] = driving_scenario_fcn(ego_state, mission, environment, driving_submode);
end

== matlab function Final_Project_PreRemoveOutputAdapter_20260527_143352/Lib_MissionManager/mission_manager_fcn ==
  data: ego_state input; active_scenario output; mission input; driving_status input; tollgate_status input; parking_status input; driving_submode output; tollgate_submode output; parking_submode output
function [active_scenario, driving_submode, tollgate_submode, parking_submode] = wrapper(ego_state, mission, driving_status, tollgate_status, parking_status)
%#codegen
% Wrapper: edit functions/mission_manager_fcn.m, NOT this block
[active_scenario, driving_submode, tollgate_submode, parking_submode] = mission_manager_fcn(ego_state, mission, driving_status, tollgate_status, parking_status);
end

== matlab function Final_Project_PreRemoveOutputAdapter_20260527_143352/Lib_Tollgate/tollgate_scenario_fcn ==
  data: ego_state input; trajectory_bus output; mission input; environment input; tollgate_submode input; target_speed output; tollgate_status output
function [trajectory_bus, target_speed, tollgate_status] = wrapper(ego_state, mission, environment, tollgate_submode)
%#codegen
% Wrapper: edit functions/tollgate_scenario_fcn.m, NOT this block
[trajectory_bus, target_speed, tollgate_status] = tollgate_scenario_fcn(ego_state, mission, environment, tollgate_submode);
end

== matlab function Final_Project_PreRemoveOutputAdapter_20260527_143352/Lib_Parking/parking_scenario_fcn ==
  data: ego_state input; trajectory_bus output; mission input; environment input; parking_submode input; target_speed output; parking_status output
function [trajectory_bus, target_speed, parking_status] = wrapper(ego_state, mission, environment, parking_submode)
%#codegen
% Wrapper: edit functions/parking_scenario_fcn.m, NOT this block
[trajectory_bus, target_speed, parking_status] = parking_scenario_fcn(ego_state, mission, environment, parking_submode);
end

== matlab function Final_Project_PreRemoveOutputAdapter_20260527_143352/Lib_VehicleController_Driving/vehicle_controller_driving_fcn ==
  data: ego_state input; steer_cmd output; active_scenario input; driving_traj input; driving_speed input; tollgate_traj input; tollgate_speed input; accel_cmd output
function [steer_cmd, accel_cmd] = wrapper(ego_state, active_scenario, driving_traj, driving_speed, tollgate_traj, tollgate_speed)
%#codegen
% Wrapper: edit functions/vehicle_controller_driving_fcn.m, NOT this block
[steer_cmd, accel_cmd] = vehicle_controller_driving_fcn(ego_state, active_scenario, driving_traj, driving_speed, tollgate_traj, tollgate_speed);
end
